simulink model "f"  (R2022b)
settings: Solver=VariableStepAuto  StartTime=0.0  StopTime=10.0  RelTol=1e-3
settings Model: Creator=AMD  LastModifiedBy=AMD

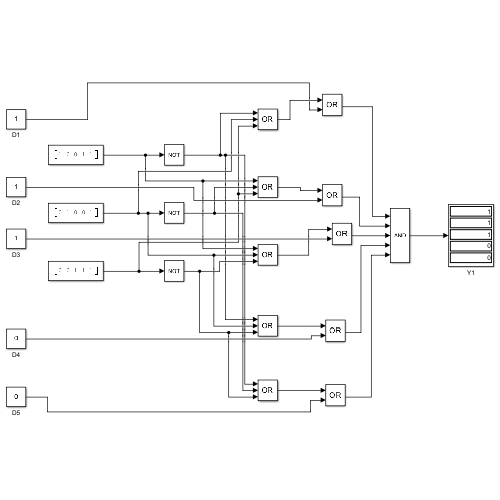
[thumbnail: Simulink's stored preview of the top-level diagram]
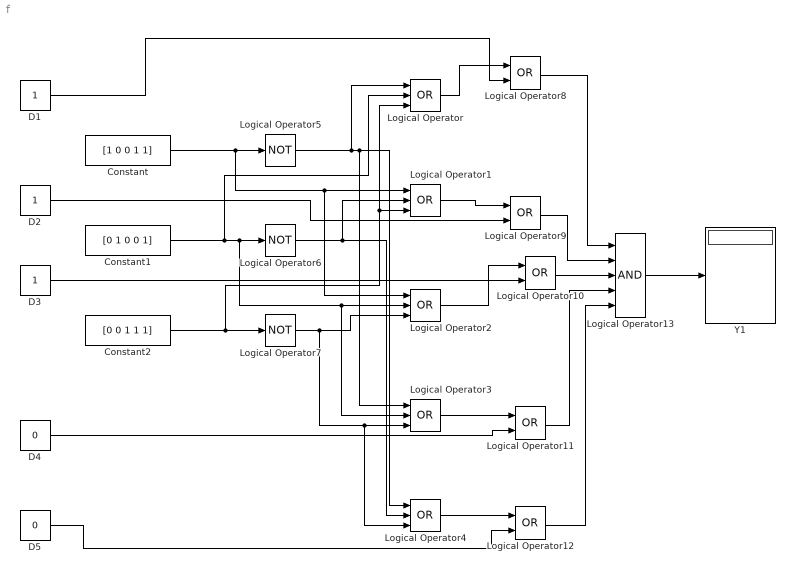
== system f ==
  Constant : Constant  Value=[1 0 0 1 1]
  Constant1 : Constant  Value=[0 1 0 0 1]
  Constant2 : Constant  Value=[0 0 1 1 1]
  D1 : Constant
  D2 : Constant
  D3 : Constant
  D4 : Constant  Value=0
  D5 : Constant  Value=0
  Logical Operator{,1..4} (5 alike) : Logic  Operator=OR  Inputs=3  AllPortsSameDT=off  OutDataTypeStr=boolean
  Logical Operator{8..12} (5 alike) : Logic  Operator=OR  AllPortsSameDT=off  OutDataTypeStr=boolean
  Logical Operator13 : Logic  Inputs=5  AllPortsSameDT=off  OutDataTypeStr=boolean
  Logical Operator5 : Logic  Operator=NOT  AllPortsSameDT=off  OutDataTypeStr=boolean
  Logical Operator6 : Logic  Operator=NOT  AllPortsSameDT=off  OutDataTypeStr=boolean
  Logical Operator7 : Logic  Operator=NOT  AllPortsSameDT=off  OutDataTypeStr=boolean
  Y1 : Display
  wires:
  Constant/1 -> Logical Operator2/1, Logical Operator1/1, Logical Operator5/1
  Logical Operator5/1 -> Logical Operator3/1, Logical Operator4/1, Logical Operator/1
  Constant1/1 -> Logical Operator/2, Logical Operator3/2, Logical Operator2/2, Logical Operator6/1
  Constant2/1 -> Logical Operator1/3, Logical Operator/3, Logical Operator7/1
  Logical Operator6/1 -> Logical Operator4/2, Logical Operator1/2
  Logical Operator7/1 -> Logical Operator4/3, Logical Operator3/3, Logical Operator2/3
  Logical Operator/1 -> Logical Operator8/1
  Logical Operator1/1 -> Logical Operator9/1
  Logical Operator2/1 -> Logical Operator10/1
  Logical Operator3/1 -> Logical Operator11/1
  Logical Operator4/1 -> Logical Operator12/1
  D5/1 -> Logical Operator12/2
  D1/1 -> Logical Operator8/2
  D2/1 -> Logical Operator9/2
  D3/1 -> Logical Operator10/2
  D4/1 -> Logical Operator11/2
  Logical Operator13/1 -> Y1/1
  Logical Operator8/1 -> Logical Operator13/1
  Logical Operator9/1 -> Logical Operator13/2
  Logical Operator10/1 -> Logical Operator13/3
  Logical Operator11/1 -> Logical Operator13/4
  Logical Operator12/1 -> Logical Operator13/5
